simulink model "pendulum_on_cart"  (R2020a)
settings: Solver=ode45  StartTime=0.0  StopTime=100  MaxStep=0.01  RelTol=1e-6
values from neighbouring files (symbols this model uses):
  alpha = @(phi) atan2(bf.delta)    [Untitled.m]    (also in butterfly_robot_phi_varphi.m = obj.m_b*obj.get_ds(varphi)*((rhoxtau + obj.J_s*obj.get_p(var; homework_5.m = @(x) cos(m_g(x)) + der_m_g(x); phase_plane.m = a(1); pplane2017b.m = (2*max(err./((abs(y)+abs(yn)+DY*1e-3)*tol)))^pow)
  beta = obj.m_b*obj.ds(phi)*(sum1*obj.diff_diff_theta(phi)-obj.tau(phi)'*obj.rho(phi)*obj.diff_theta(phi)^2+sum2*obj.dds(phi))    [butterfly_robot.m]    (also in butterfly_robot_phi_varphi.m = obj.m_b*obj.get_ds(varphi)*((rhoxtau+obj.J_s*obj.get_p(varph; homework_5.m = @(x) sec_der_m_g(x); phase_plane.m = a(2))
  controller = @(x,dx,x_star,dx_star,time,transverse) epsilon(x_star,transverse(2),dx_star,transverse(3)) + psi(x_star,transverse(2))*v(x,dx,time,transverse)    [homework_5.m]
  dx_0 = 0.2    [homework_5.m]
  f_ddx = matlabFunction(poly2sym(f))    [homework_5.m]
  f_dx = matlabFunction(poly2sym(f))    [homework_5.m]
  f_x = matlabFunction(poly2sym(f))    [homework_5.m]
  func_A = @(t) A(f_x(t),f_dx(t),f_ddx(t))    [homework_5.m]
  func_B = @(t) B(f_x(t),f_dx(t))    [homework_5.m]
  interpolation_for_X = @(x)[interp1(phi,reshape(X(1,1,:),1,length(X)),x) interp1(phi,reshape(X(1,2,:),1,length(X)),x) interp1(phi,reshape(X(1,3,:),1,length(X)),x) interp1(phi,reshape(X(1,4,:),1,length(X)),x) ... (first row only)    [butterfly_robot.m]    (also in butterfly_robot_phi_varphi.m = @(x)[interp1(phi,reshape(X(1,1,:),1,length(X)),x) interp1(ph; homework_5.m = @(x)[interp1(time,reshape(X(1,1,:),1,length(X)),x) interp1(t)
  L = [1 obj.diff_theta(q(2)) ... (first row only)    [butterfly_robot.m]    (also in butterfly_robot_phi_varphi.m = [1 obj.get_dtheta(q(2)); homework_5.m = -1.3; pplane2017b.m = length(t))
  v = @(x,dx,time,transverse) -(1/Gamma)*B(x,dx)'*interpolation_for_X(mod(time,time(end)))*transverse    [homework_5.m]    (also in phase_plane.m = zeros(size(x)); pplane2017b.m = [ud.rr,rr])
  W = @(x,y,ddx,ddx_star,v)-g*(sin(m_g(x))+sin(y+m_g(x)))-(-cos(m_g(x))+cos(y+m_g(x)))*ddx-v    [homework_5.m]
  y = @(theta, x) theta - m_g(x)    [homework_5.m]    (also in jalla_lqr.m = states; pplane2017b.m = y + h*(s1 + 2*s2 + 2*s3 +s4)/6)
  y_dot = @(theta_dot , x, dx) theta_dot - der_m_g(x)*dx    [homework_5.m]
libraries: simulink x2
settings Model: Creator=g-oft  LastModifiedBy=g-oft

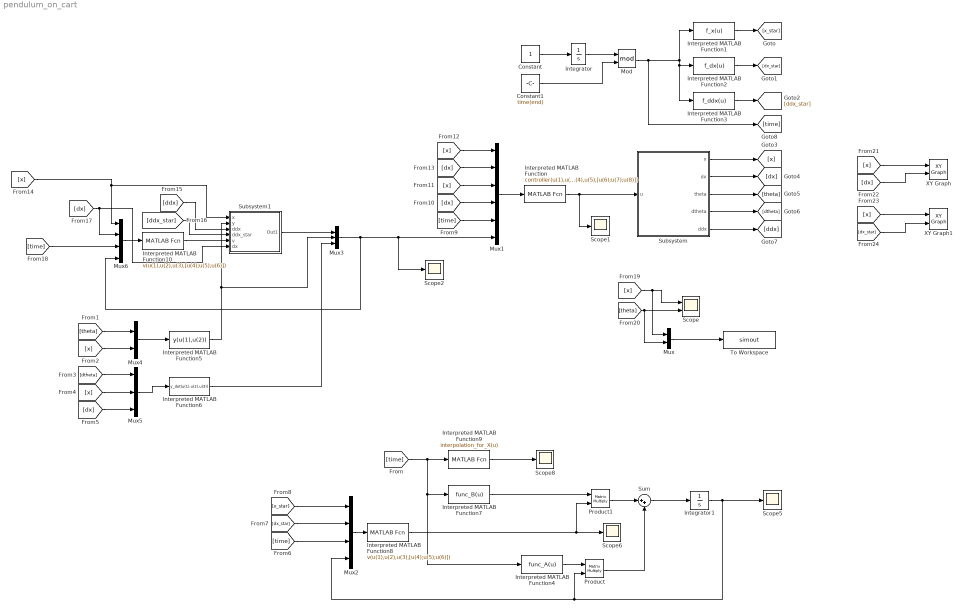
== system pendulum_on_cart ==
  Constant : Constant
  Constant1 : Constant  Value=time(end)
  Integrator : Integrator
  Integrator1 : Integrator  InitialCondition=[0;0.01;0]
  Interpreted MATLAB Function : MATLABFcn  MATLABFcn=controller(u(1),u(2),u(3),u(4),u(5),[u(6);u(7);u(8)])  OutputDimensions=1  Output1D=off
  Interpreted MATLAB Function1 : MATLABFcn  MATLABFcn=f_x(u)
  Interpreted MATLAB Function10 : MATLABFcn  MATLABFcn=v(u(1),u(2),u(3),[u(4);u(5);u(6)])  OutputDimensions=1  Output1D=off
  Interpreted MATLAB Function2 : MATLABFcn  MATLABFcn=f_dx(u)
  Interpreted MATLAB Function3 : MATLABFcn  MATLABFcn=f_ddx(u)
  Interpreted MATLAB Function4 : MATLABFcn  MATLABFcn=func_A(u)  Output1D=off
  Interpreted MATLAB Function5 : MATLABFcn  MATLABFcn=y(u(1),u(2))  OutputDimensions=1  Output1D=off
  Interpreted MATLAB Function6 : MATLABFcn  MATLABFcn=y_dot(u(1),u(2),u(3))  OutputDimensions=1  Output1D=off
  Interpreted MATLAB Function7 : MATLABFcn  MATLABFcn=func_B(u)
  Interpreted MATLAB Function8 : MATLABFcn  MATLABFcn=v(u(1),u(2),u(3),[u(4);u(5);u(6)])  Output1D=off
  Interpreted MATLAB Function9 : MATLABFcn  MATLABFcn=interpolation_for_X(u)
  Mod : Math  Operator=mod  SaturateOnIntegerOverflow=on
  Mux : Mux  Inputs=2
  Mux1 : Mux  Inputs=6
  Mux2 : Mux
  Mux3 : Mux  Inputs=3
  Mux4 : Mux  Inputs=2
  Mux5 : Mux  Inputs=3
  Mux6 : Mux
  Product : Product  Multiplication=Matrix(*)
  Product1 : Product  Multiplication=Matrix(*)
  Scope : Scope  NumInputPorts=2
  Scope{1..2,5..6,8} (5 alike) : Scope
  Subsystem : Subsystem
  Subsystem1 : Subsystem
  Sum : Sum  Inputs=|++
  To Workspace : ToWorkspace  VariableName=simout  SampleTime=-1
  XY Graph : simulink/Sinks/XY Graph  xmin=-1  xmax=1  ymin=-1  ymax=1  st=-1
  XY Graph1 : simulink/Sinks/XY Graph  xmin=-1  xmax=1  ymin=-1  ymax=1  st=-1
  wires:
  Mux/1 -> To Workspace/1
  Interpreted MATLAB Function/1 -> Scope1/1, Subsystem/1(u)
  Mux1/1 -> Interpreted MATLAB Function/1
  Constant/1 -> Integrator/1
  Interpreted MATLAB Function5/1 -> Mux3/2, Subsystem1/2(y)
  Mux4/1 -> Interpreted MATLAB Function5/1
  Mux5/1 -> Interpreted MATLAB Function6/1
  Interpreted MATLAB Function4/1 -> Product/1
  Product/1 -> Sum/2
  Interpreted MATLAB Function7/1 -> Product1/1
  Sum/1 -> Integrator1/1
  Integrator1/1 -> Scope5/1, Mux2/4, Product/2
  Interpreted MATLAB Function8/1 -> Product1/2, Scope6/1
  Mod/1 -> [time], Interpreted MATLAB Function3/1, Interpreted MATLAB Function2/1, Interpreted MATLAB Function1/1
  Mux2/1 -> Interpreted MATLAB Function8/1
  Product1/1 -> Sum/1
  Interpreted MATLAB Function9/1 -> Scope8/1
  Integrator/1 -> Mod/1
  Constant1/1 -> Mod/2
  Interpreted MATLAB Function10/1 -> Subsystem1/5(v)
  Interpreted MATLAB Function3/1 -> [ddx_star]
  Interpreted MATLAB Function2/1 -> [dx_star]
  Interpreted MATLAB Function1/1 -> [x_star]
  Subsystem/2(dx) -> [dx]
  Subsystem/3(theta) -> [theta]
  Subsystem/4(dtheta) -> [dtheta]
  Subsystem/5(ddx) -> [ddx]
  [time] -> Interpreted MATLAB Function7/1, Interpreted MATLAB Function4/1, Interpreted MATLAB Function9/1
  Subsystem1/1(Out1) -> Mux3/1
  Interpreted MATLAB Function6/1 -> Mux3/3
  Mux3/1 -> Mux6/4, Scope2/1, Mux1/6
  [theta] -> Mux4/1
  [x] -> Mux4/2
  [dtheta] -> Mux5/1
  [x] -> Mux5/2
  [dx] -> Mux5/3
  [time] -> Mux2/3
  [dx_star] -> Mux2/2
  [x_star] -> Mux2/1
  [time] -> Mux1/5
  [x] -> Mux1/3
  [dx] -> Mux1/4
  [x] -> Mux1/1
  [dx] -> Mux1/2
  [x] -> Mux6/1, Subsystem1/1(x)
  [ddx] -> Subsystem1/3(ddx)
  [ddx_star] -> Subsystem1/4(ddx_star)
  [dx] -> Mux6/2, Subsystem1/6(dx)
  Mux6/1 -> Interpreted MATLAB Function10/1
  [time] -> Mux6/3
  [x] -> Mux/1, Scope/1
  [theta] -> Mux/2, Scope/2
  [x] -> XY Graph/1
  [dx] -> XY Graph/2
  [x] -> XY Graph1/1
  [dx_star] -> XY Graph1/2
  Subsystem/1(x) -> [x]

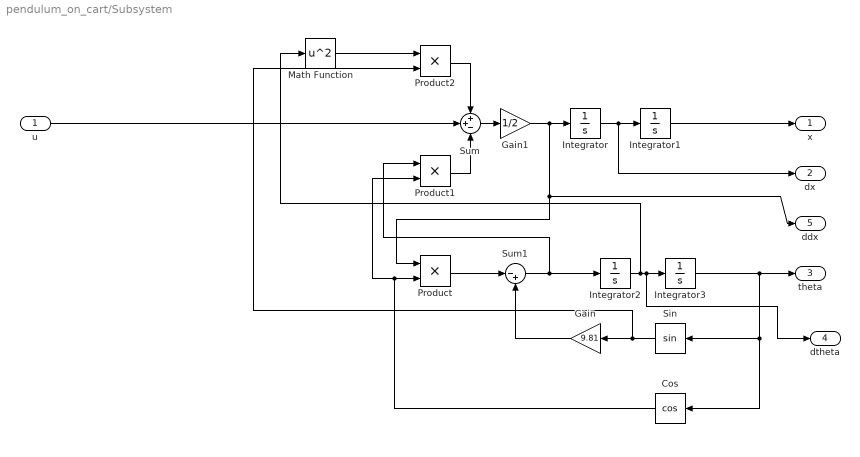
== system pendulum_on_cart/Subsystem ==
  u : Inport
  Cos : Trigonometry  Operator=cos
  Gain : Gain  Gain=9.81
  Gain1 : Gain  Gain=1/2
  Integrator : Integrator  InitialCondition=dx_0
  Integrator1 : Integrator
  Integrator2 : Integrator  InitialCondition=(1+L)*dx_0
  Integrator3 : Integrator
  Math Function : Math  Operator=square  SaturateOnIntegerOverflow=on
  Product : Product
  Product1 : Product
  Product2 : Product
  Sin : Trigonometry
  Sum : Sum  Inputs=++-
  Sum1 : Sum  Inputs=|-+
  x : Outport
  dx : Outport  Port=2
  theta : Outport  Port=3
  dtheta : Outport  Port=4
  ddx : Outport  Port=5
  wires:
  Sum1/1 -> Product1/1, Integrator2/1
  u/1 -> Sum/2
  Cos/1 -> Product1/2, Product/2
  Product2/1 -> Sum/1
  Gain/1 -> Sum1/2
  Product1/1 -> Sum/3
  Product/1 -> Sum1/1
  Sum/1 -> Gain1/1
  Sin/1 -> Product2/2, Gain/1
  Integrator2/1 -> dtheta/1, Integrator3/1, Math Function/1
  Math Function/1 -> Product2/1
  Integrator3/1 -> theta/1, Cos/1, Sin/1
  Gain1/1 -> Product/1, ddx/1, Integrator/1
  Integrator1/1 -> x/1
  Integrator/1 -> dx/1, Integrator1/1

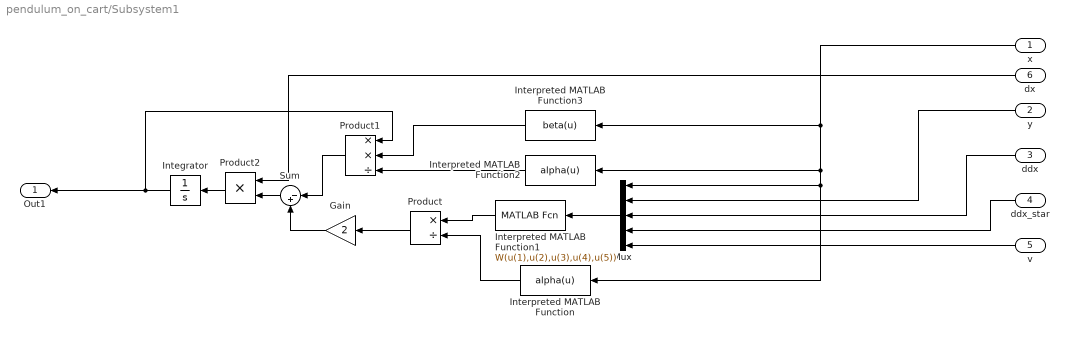
== system pendulum_on_cart/Subsystem1 ==
  x : Inport
  y : Inport  Port=2
  ddx : Inport  Port=3
  ddx_star : Inport  Port=4
  v : Inport  Port=5
  dx : Inport  Port=6
  Gain : Gain  Gain=2
  Integrator : Integrator
  Interpreted MATLAB Function : MATLABFcn  MATLABFcn=alpha(u)
  Interpreted MATLAB Function1 : MATLABFcn  MATLABFcn=W(u(1),u(2),u(3),u(4),u(5))
  Interpreted MATLAB Function2 : MATLABFcn  MATLABFcn=alpha(u)
  Interpreted MATLAB Function3 : MATLABFcn  MATLABFcn=beta(u)
  Mux : Mux  Inputs=5
  Product : Product  Inputs=*/
  Product1 : Product  Inputs=**/
  Product2 : Product
  Sum : Sum  Inputs=|-+
  Out1 : Outport
  wires:
  Integrator/1 -> Out1/1, Product1/1
  Mux/1 -> Interpreted MATLAB Function1/1
  x/1 -> Interpreted MATLAB Function2/1, Interpreted MATLAB Function/1, Mux/1, Interpreted MATLAB Function3/1
  y/1 -> Mux/2
  ddx/1 -> Mux/3
  ddx_star/1 -> Mux/4
  v/1 -> Mux/5
  Interpreted MATLAB Function1/1 -> Product/1
  Product/1 -> Gain/1
  Interpreted MATLAB Function/1 -> Product/2
  Gain/1 -> Sum/2
  Interpreted MATLAB Function2/1 -> Product1/3
  Interpreted MATLAB Function3/1 -> Product1/2
  Product1/1 -> Sum/1
  Sum/1 -> Product2/2
  Product2/1 -> Integrator/1
  dx/1 -> Product2/1
